simulink model "modelo_gemelo_digital"  (R2026a)
settings: Solver=ode45  StopTime=58999
libraries: simulink x3
settings Model: SimulationMode=rapid-accelerator

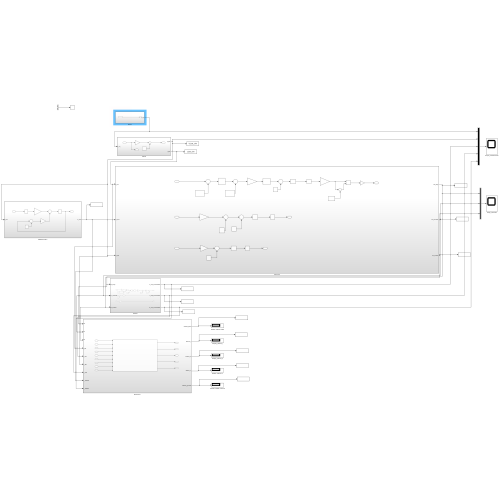
[thumbnail: Simulink's stored preview of the top-level diagram]
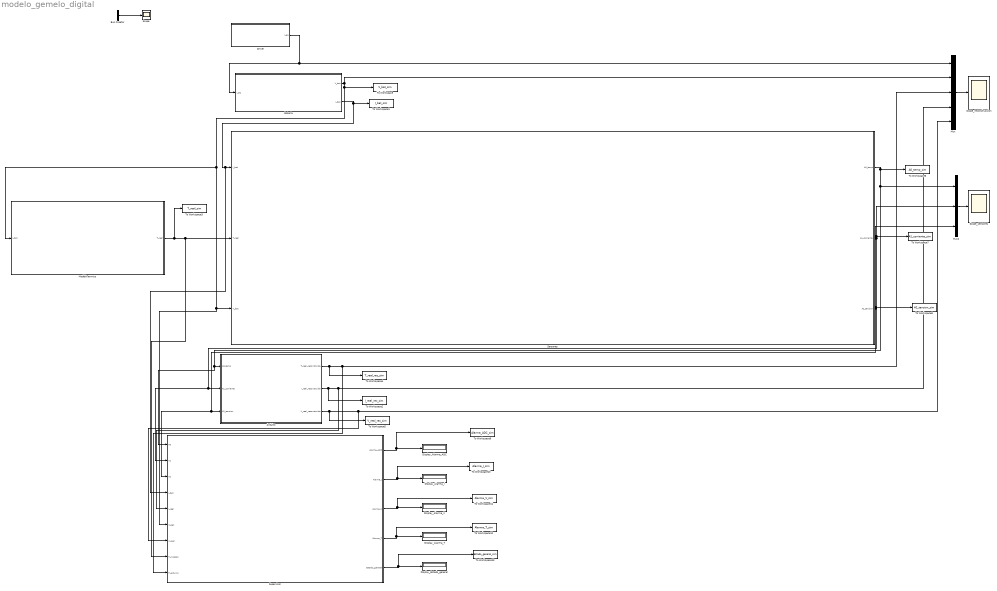
== system modelo_gemelo_digital ==
  Arduino : Subsystem
  Bateria : Subsystem
  Bus Creator : BusCreator  Inputs=2
  Display_Alarma_ADC : Display
  Display_Alarma_I : Display
  Display_Alarma_T : Display
  Display_Alarma_V : Display
  Display_Estado_general : Display
  Driver : Subsystem
  ModeloTermico : Subsystem
  Mux : Mux  Inputs=5
  Mux2 : Mux  Inputs=3
  Scope : Scope
      settings: ActiveDisplayYMinimum=32.397318000944054  ActiveDisplayYMaximum=32.413714810160194
  Scope_reconstruccion : Scope
      settings: ActiveDisplayYMinimum=-9.0542521994134866  ActiveDisplayYMaximum=58.516617790811338
  Scope_sensores : Scope
      settings: ActiveDisplayYMinimum=1.3440860215053765  ActiveDisplayYMaximum=5.9384164222873892  DataLoggingVariableName=ScopeData3
  Sensores : Subsystem
  Supervisor : Subsystem
  To Workspace : ToWorkspace  VariableName=V_bat_sim  SaveFormat=Timeseries  SampleTime=-1
  To Workspace1 : ToWorkspace  VariableName=I_bat_sim  SaveFormat=Timeseries  SampleTime=-1
  To Workspace10 : ToWorkspace  VariableName=Alarma_I_sim  SaveFormat=Timeseries  SampleTime=-1
  To Workspace11 : ToWorkspace  VariableName=Alarma_V_sim  SaveFormat=Timeseries  SampleTime=-1
  To Workspace12 : ToWorkspace  VariableName=Alarma_T_sim  SaveFormat=Timeseries  SampleTime=-1
  To Workspace13 : ToWorkspace  VariableName=Estado_general_sim  SaveFormat=Timeseries  SampleTime=-1
  To Workspace2 : ToWorkspace  VariableName=I_real_rec_sim  SaveFormat=Timeseries  SampleTime=-1
  To Workspace3 : ToWorkspace  VariableName=T_real_sim  SaveFormat=Timeseries  SampleTime=-1
  To Workspace4 : ToWorkspace  VariableName=T_real_rec_sim  SaveFormat=Timeseries  SampleTime=-1
  To Workspace5 : ToWorkspace  VariableName=V_real_rec_sim  SaveFormat=Timeseries  SampleTime=-1
  To Workspace6 : ToWorkspace  VariableName=A0_temp_sim  SaveFormat=Timeseries  SampleTime=-1
  To Workspace7 : ToWorkspace  VariableName=A1_corriente_sim  SaveFormat=Timeseries  SampleTime=-1
  To Workspace8 : ToWorkspace  VariableName=A2_tension_sim  SaveFormat=Timeseries  SampleTime=-1
  To Workspace9 : ToWorkspace  VariableName=Alarma_ADC_sim  SaveFormat=Timeseries  SampleTime=-1
  wires:
  Driver/1(I_eq) -> Mux/1, Bateria/1(I_eq)
  Mux/1 -> Scope_reconstruccion/1
  Arduino/1(T_real_reconstruida) -> To Workspace4/1, Supervisor/9(T_arduino), Mux/3
  Arduino/3(V_real_reconstruida) -> To Workspace5/1, Supervisor/7(V_real), Mux/5
  Sensores/1(A0_temp) -> To Workspace6/1, Mux2/1, Arduino/1(A0_temp), Supervisor/1(A0)
  Sensores/2(A1_corriente) -> Mux2/2, To Workspace7/1, Arduino/2(A1_corriente), Supervisor/2(A1)
  Sensores/3(A2_tension) -> To Workspace8/1, Mux2/3, Arduino/3(A2_tension), Supervisor/3(A2)
  Bateria/2(I_bat) -> To Workspace1/1, Supervisor/4(I_bat), Sensores/1(I_bat)
  ModeloTermico/1(T_real) -> To Workspace3/1, Sensores/2(T_real), Supervisor/8(T_modelo)
  Bateria/1(V_bat) -> To Workspace/1, ModeloTermico/1(I_bat), Sensores/3(V_bat), Supervisor/6(V_bat), Mux/2
  Mux2/1 -> Scope_sensores/1
  Supervisor/1(Alarma_ADC) -> To Workspace9/1, Display_Alarma_ADC/1
  Supervisor/2(Alarma_I) -> To Workspace10/1, Display_Alarma_I/1
  Supervisor/3(Alarma_V) -> To Workspace11/1, Display_Alarma_V/1
  Supervisor/4(Alarma_T) -> To Workspace12/1, Display_Alarma_T/1
  Supervisor/5(Estado_general) -> To Workspace13/1, Display_Estado_general/1
  Arduino/2(I_real_reconstruida) -> To Workspace2/1, Supervisor/5(I_real), Mux/4
  Bus Creator/1 -> Scope/1

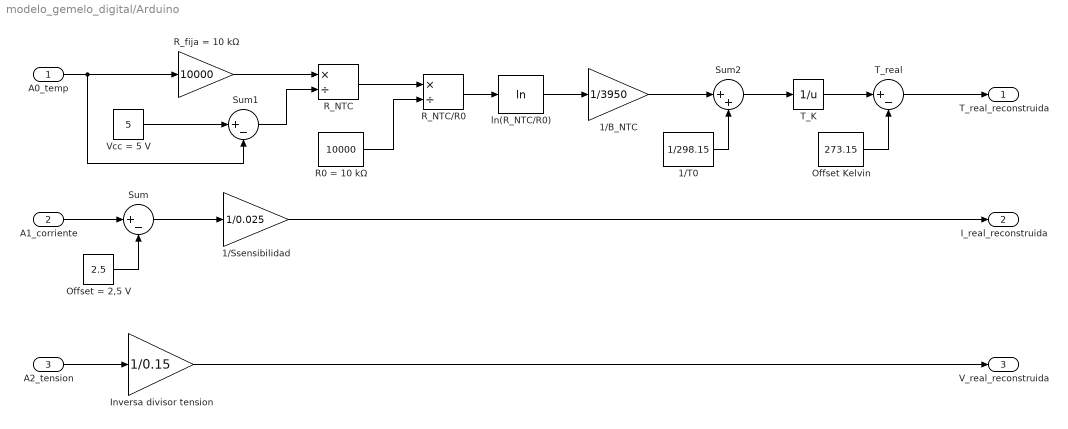
== system modelo_gemelo_digital/Arduino ==
  A0_temp : Inport
  A1_corriente : Inport  Port=2
  A2_tension : Inport  Port=3
  1/B_NTC : Gain  Gain=1/3950
  1/Ssensibilidad : Gain  Gain=1/0.025
  1/T0 : Constant  Value=1/298.15
  Inversa divisor tension : Gain  Gain=1/0.15
  Offset = 2,5 V : Constant  Value=2.5
  Offset Kelvin : Constant  Value=273.15
  R0 = 10 kΩ : Constant  Value=10000
  R_NTC : Product  Inputs=*/
  R_NTC/R0 : Product  Inputs=*/
  R_fija = 10 kΩ : Gain  Gain=10000
  Sum : Sum  Inputs=|+-
  Sum1 : Sum  Inputs=|+-
  Sum2 : Sum  Inputs=|++
  T_K : Math  Operator=reciprocal
  T_real : Sum  Inputs=|+-
  Vcc = 5 V : Constant  Value=5
  ln(R_NTC/R0) : Math  Operator=log
  T_real_reconstruida : Outport
  I_real_reconstruida : Outport  Port=2
  V_real_reconstruida : Outport  Port=3
  wires:
  A2_tension/1 -> Inversa divisor tension/1
  Offset = 2,5 V/1 -> Sum/2
  Sum/1 -> 1/Ssensibilidad/1
  Vcc = 5 V/1 -> Sum1/1
  A1_corriente/1 -> Sum/1
  A0_temp/1 -> R_fija = 10 kΩ/1, Sum1/2
  R_NTC/1 -> R_NTC/R0/1
  R0 = 10 kΩ/1 -> R_NTC/R0/2
  R_NTC/R0/1 -> ln(R_NTC/R0)/1
  ln(R_NTC/R0)/1 -> 1/B_NTC/1
  1/B_NTC/1 -> Sum2/1
  1/T0/1 -> Sum2/2
  Sum2/1 -> T_K/1
  T_K/1 -> T_real/1
  Offset Kelvin/1 -> T_real/2
  T_real/1 -> T_real_reconstruida/1
  1/Ssensibilidad/1 -> I_real_reconstruida/1
  Inversa divisor tension/1 -> V_real_reconstruida/1
  R_fija = 10 kΩ/1 -> R_NTC/1
  Sum1/1 -> R_NTC/2

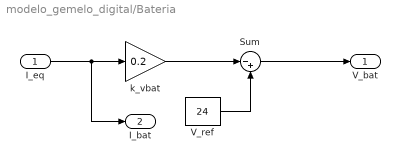
== system modelo_gemelo_digital/Bateria ==
  I_eq : Inport
  Sum : Sum  Inputs=|-+
  V_ref : Constant  Value=24
  k_vbat : Gain  Gain=0.2
  V_bat : Outport
  I_bat : Outport  Port=2
  wires:
  V_ref/1 -> Sum/2
  I_eq/1 -> I_bat/1, k_vbat/1
  k_vbat/1 -> Sum/1
  Sum/1 -> V_bat/1

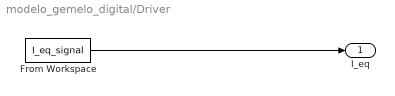
== system modelo_gemelo_digital/Driver ==
  From Workspace : FromWorkspace  VariableName=I_eq_signal
  I_eq : Outport
  wires:
  From Workspace/1 -> I_eq/1

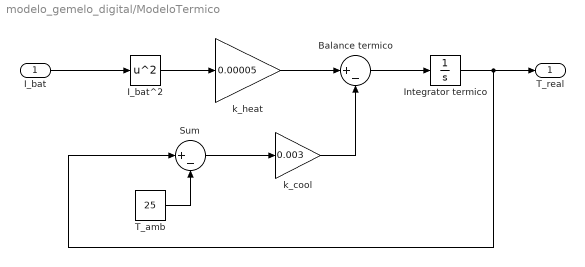
== system modelo_gemelo_digital/ModeloTermico ==
  I_bat : Inport
  Balance termico : Sum  Inputs=|+-
  I_bat^2 : Math  Operator=square
  Integrator termico : Integrator  InitialCondition=25
  Sum : Sum  Inputs=|+-
  T_amb : Constant  Value=25
  k_cool : Gain  Gain=0.003
  k_heat : Gain  Gain=0.00005
  T_real : Outport
  wires:
  T_amb/1 -> Sum/2
  Sum/1 -> k_cool/1
  I_bat/1 -> I_bat^2/1
  k_cool/1 -> Balance termico/2
  Integrator termico/1 -> T_real/1, Sum/1
  I_bat^2/1 -> k_heat/1
  Balance termico/1 -> Integrator termico/1
  k_heat/1 -> Balance termico/1

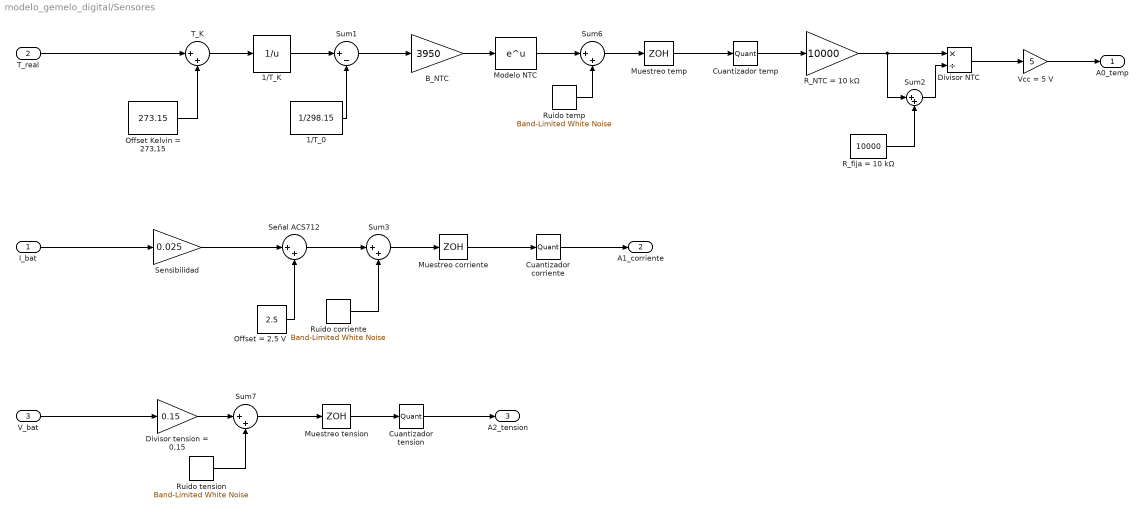
== system modelo_gemelo_digital/Sensores ==
  I_bat : Inport
  T_real : Inport  Port=2
  V_bat : Inport  Port=3
  1/T_0 : Constant  Value=1/298.15
  1/T_K : Math  Operator=reciprocal
  B_NTC : Gain  Gain=3950
  Cuantizador corriente : Quantizer  QuantizationInterval=5/1023
  Cuantizador temp : Quantizer  QuantizationInterval=5/1023
  Cuantizador tension : Quantizer  QuantizationInterval=5/1023
  Divisor NTC : Product  Inputs=*/
  Divisor tension = 0,15 : Gain  Gain=0.15
  Modelo NTC : Math
  Muestreo corriente : ZeroOrderHold  SampleTime=0.01
  Muestreo temp : ZeroOrderHold  SampleTime=0.01
  Muestreo tension : ZeroOrderHold  SampleTime=0.01
  Offset = 2,5 V : Constant  Value=2.5
  Offset Kelvin = 273,15 : Constant  Value=273.15
  R_NTC = 10 kΩ : Gain  Gain=10000
  R_fija = 10 kΩ : Constant  Value=10000
  Ruido corriente : simulink/Sources/Band-Limited White Noise  Cov=1e-6  Ts=0.01  seed=[23341]
  Ruido temp : simulink/Sources/Band-Limited White Noise  Cov=1e-6  Ts=0.01  seed=[23341]
  Ruido tension : simulink/Sources/Band-Limited White Noise  Cov=1e-6  Ts=0.01  seed=[23341]
  Sensibilidad : Gain  Gain=0.025
  Señal ACS712 : Sum  Inputs=|++
  Sum1 : Sum  Inputs=|+-
  Sum{2..3,6..7} (4 alike) : Sum  Inputs=|++
  T_K : Sum  Inputs=|++
  Vcc = 5 V : Gain  Gain=5
  A0_temp : Outport
  A1_corriente : Outport  Port=2
  A2_tension : Outport  Port=3
  wires:
  Sum3/1 -> Muestreo corriente/1
  Muestreo tension/1 -> Cuantizador tension/1
  Sensibilidad/1 -> Señal ACS712/1
  1/T_K/1 -> Sum1/1
  Offset = 2,5 V/1 -> Señal ACS712/2
  Sum6/1 -> Muestreo temp/1
  Muestreo temp/1 -> Cuantizador temp/1
  Sum1/1 -> B_NTC/1
  1/T_0/1 -> Sum1/2
  Señal ACS712/1 -> Sum3/1
  Sum7/1 -> Muestreo tension/1
  T_K/1 -> 1/T_K/1
  Offset Kelvin = 273,15/1 -> T_K/2
  Muestreo corriente/1 -> Cuantizador corriente/1
  Ruido tension/1 -> Sum7/2
  Divisor tension = 0,15/1 -> Sum7/1
  Ruido corriente/1 -> Sum3/2
  Ruido temp/1 -> Sum6/2
  B_NTC/1 -> Modelo NTC/1
  T_real/1 -> T_K/1
  I_bat/1 -> Sensibilidad/1
  V_bat/1 -> Divisor tension = 0,15/1
  Modelo NTC/1 -> Sum6/1
  Cuantizador temp/1 -> R_NTC = 10 kΩ/1
  Cuantizador tension/1 -> A2_tension/1
  Cuantizador corriente/1 -> A1_corriente/1
  R_NTC = 10 kΩ/1 -> Sum2/1, Divisor NTC/1
  R_fija = 10 kΩ/1 -> Sum2/2
  Sum2/1 -> Divisor NTC/2
  Divisor NTC/1 -> Vcc = 5 V/1
  Vcc = 5 V/1 -> A0_temp/1

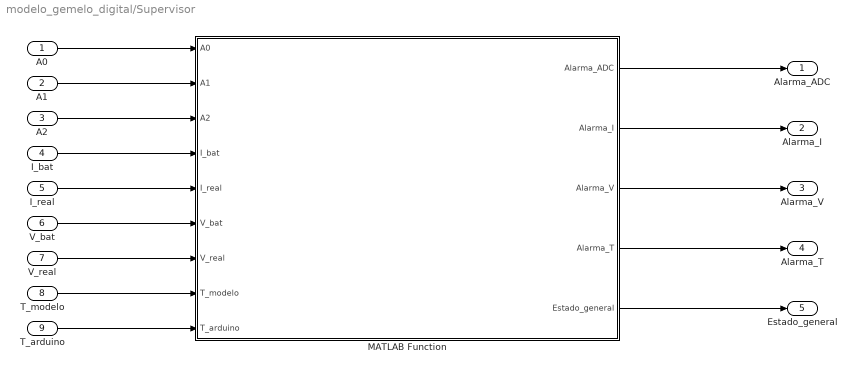
== system modelo_gemelo_digital/Supervisor ==
  A0 : Inport
  A1 : Inport  Port=2
  A2 : Inport  Port=3
  I_bat : Inport  Port=4
  I_real : Inport  Port=5
  V_bat : Inport  Port=6
  V_real : Inport  Port=7
  T_modelo : Inport  Port=8
  T_arduino : Inport  Port=9
  MATLAB Function : MATLAB Function  TreatAsAtomicUnit=on
  Alarma_ADC : Outport
  Alarma_I : Outport  Port=2
  Alarma_V : Outport  Port=3
  Alarma_T : Outport  Port=4
  Estado_general : Outport  Port=5
  wires:
  A0/1 -> MATLAB Function/1(A0)
  A1/1 -> MATLAB Function/2(A1)
  A2/1 -> MATLAB Function/3(A2)
  I_bat/1 -> MATLAB Function/4(I_bat)
  V_bat/1 -> MATLAB Function/6(V_bat)
  I_real/1 -> MATLAB Function/5(I_real)
  V_real/1 -> MATLAB Function/7(V_real)
  T_arduino/1 -> MATLAB Function/9(T_arduino)
  T_modelo/1 -> MATLAB Function/8(T_modelo)
  MATLAB Function/1(Alarma_ADC) -> Alarma_ADC/1
  MATLAB Function/2(Alarma_I) -> Alarma_I/1
  MATLAB Function/3(Alarma_V) -> Alarma_V/1
  MATLAB Function/4(Alarma_T) -> Alarma_T/1
  MATLAB Function/5(Estado_general) -> Estado_general/1

== matlab function modelo_gemelo_digital/Supervisor/MATLAB Function ==
  data: A0 input; Alarma_ADC output; A1 input; A2 input; I_bat input; I_real input; V_bat input; V_real input; T_modelo input; T_arduino input; Alarma_I output; Alarma_V output; Alarma_T output; Estado_general output
function [Alarma_ADC, Alarma_I, Alarma_V, Alarma_T, Estado_general] = Modulo_Supervisor(A0,A1,A2,I_bat,I_real,V_bat,V_real,T_modelo,T_arduino)

% Supervisor de estado del gemelo digital
% Estado_general:
% 0 = Normal
% 1 = Aviso
% 2 = Critico

%% Umbrales

I_umbral = 2;        % A
V_umbral = 1;        % V
T_aviso = 40;        % ºC
T_critico = 50;      % ºC

%% Alarma por rango ADC Arduino

Alarma_ADC = 0;

if A0 < 0 || A0 > 5 || A1 < 0 || A1 > 5 || A2 < 0 || A2 > 5
    Alarma_ADC = 1;
end

%% Alarma por error de corriente

Alarma_I = 0;

if abs(I_bat - I_real) > I_umbral
    Alarma_I = 1;
end

%% Alarma por error de tensión

Alarma_V = 0;

if abs(V_bat - V_real) > V_umbral
    Alarma_V = 1;
end

%% Alarma térmica

Alarma_T = 0;

if T_modelo > T_aviso || T_arduino > T_aviso
    Alarma_T = 1;
end

%% Estado general

Estado_general = 0;

% Condición crítica:
% - señales analógicas fuera de rango
% - temperatura muy alta
if Alarma_ADC == 1 || T_modelo > T_critico || T_arduino > T_critico
    Estado_general = 2;

    % Condición de aviso:
    % - error de corriente
    % - error de tensión
    % - temperatura en aviso
elseif Alarma_I == 1 || Alarma_V == 1 || Alarma_T == 1
    Estado_general = 1;

    % Sin alarmas
else
    Estado_general = 0;
end
